simulink model "hw3_1b"  (R2025b)
settings: Solver=VariableStepAuto  StartTime=0.0  StopTime=20  RelTol=1e-3
settings Model: Creator=stand  LastModifiedBy=stand

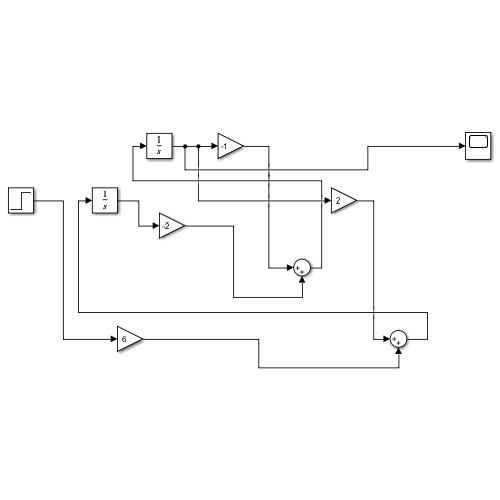
[thumbnail: Simulink's stored preview of the top-level diagram]
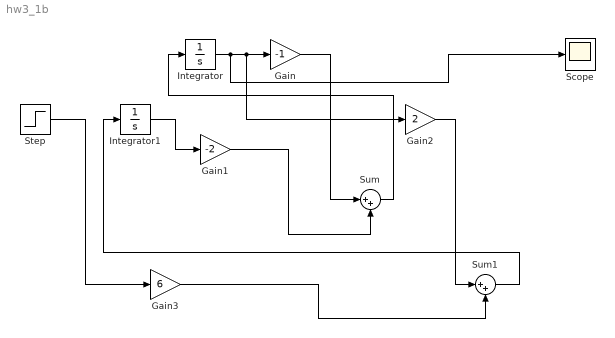
== system hw3_1b ==
  Gain : Gain  Gain=-1
  Gain1 : Gain  Gain=-2
  Gain2 : Gain  Gain=2
  Gain3 : Gain  Gain=6
  Integrator : Integrator
  Integrator1 : Integrator
  Scope : Scope
  Step : Step  Time=0  SampleTime=0
  Sum : Sum  Inputs=|++
  Sum1 : Sum  Inputs=|++
  wires:
  Gain1/1 -> Sum/2
  Integrator/1 -> Scope/1, Gain2/1, Gain/1
  Integrator1/1 -> Gain1/1
  Gain/1 -> Sum/1
  Step/1 -> Gain3/1
  Gain2/1 -> Sum1/1
  Gain3/1 -> Sum1/2
  Sum/1 -> Integrator/1
  Sum1/1 -> Integrator1/1
